simulink model "ardupilotsailboat"  (R2024a)
settings: Solver=ode15s  StartTime=0.0  StopTime=2  RelTol=1e-3
values from neighbouring files (symbols this model uses):
  Ixx = 1/120 * pi * rho * L * B * T * (4*T^2 + B^2)    (= 0.835683076278)    [parameterCalculations.m]
  Izz = 1/120 * pi * rho * L * B * T * (B^2 + L^2)    (= 1.17027496573)    [parameterCalculations.m]
  m = 2.7    [parameterCalculations.m]
  m11 = m*k11    [parameterCalculations.m]
  m22 = m*k22    [parameterCalculations.m]
  m24 = 0    [parameterCalculations.m]
  m26 = xb*m22    [parameterCalculations.m]
  m66 = k66*Izz    [parameterCalculations.m]
  Nr = -pi * T^2/L^2 * (0.25 +0.039 * B/T - 0.56 * B/L)    (= -0.104988463049)    [parameterCalculations.m]
  Nv = -pi * T^2/L^2 * (0.5 +2.4 * T/L)    (= -0.841300100031)    [parameterCalculations.m]
  Yv = -pi * T^2/L^2 * (1 +0.4 * CB * B/T)    (= -0.560439243466)    [parameterCalculations.m]
undefined symbols (not defined in the file or in its folder): Waypoints
libraries: cstblocks x6, simulink x4, vrlib x1
(part 2 of 2)

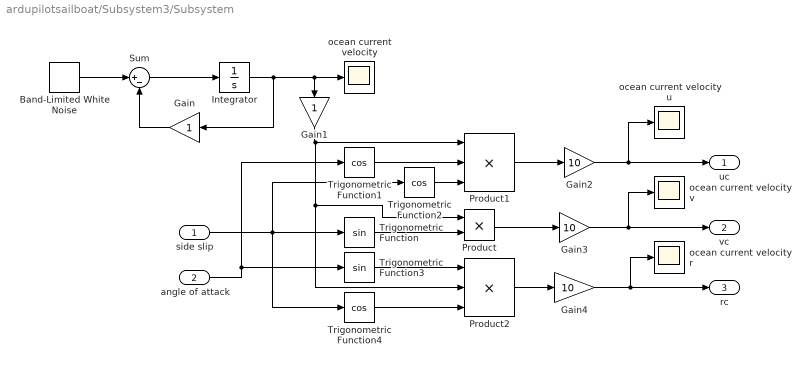
== system ardupilotsailboat/Subsystem3/Subsystem ==
  side slip : Inport
  angle of attack : Inport  Port=2
  Band-Limited White Noise : simulink/Sources/Band-Limited White Noise  Cov=[0.03]  Ts=1  seed=[23341]
  Gain : Gain
  Gain1 : Gain
  Gain2 : Gain  Gain=10
  Gain3 : Gain  Gain=10
  Gain4 : Gain  Gain=10
  Integrator : Integrator
  Product : Product
  Product1 : Product  Inputs=3
  Product2 : Product  Inputs=3
  Sum : Sum  Inputs=|+-
  Trigonometric Function : Trigonometry
  Trigonometric Function1 : Trigonometry  Operator=cos
  Trigonometric Function2 : Trigonometry  Operator=cos
  Trigonometric Function3 : Trigonometry
  Trigonometric Function4 : Trigonometry  Operator=cos
  ocean current velocity : Scope
  ocean current velocity r : Scope
  ocean current velocity u : Scope
  ocean current velocity v : Scope
  uc : Outport
  vc : Outport  Port=2
  rc : Outport  Port=3
  wires:
  Sum/1 -> Integrator/1
  Band-Limited White Noise/1 -> Sum/1
  Integrator/1 -> ocean current velocity/1, Gain1/1, Gain/1
  Gain/1 -> Sum/2
  Trigonometric Function/1 -> Product/2
  side slip/1 -> Trigonometric Function4/1, Trigonometric Function2/1, Trigonometric Function/1
  Product/1 -> Gain3/1
  Trigonometric Function2/1 -> Product1/3
  Trigonometric Function1/1 -> Product1/2
  Product1/1 -> Gain2/1
  Trigonometric Function3/1 -> Product2/1
  Trigonometric Function4/1 -> Product2/3
  angle of attack/1 -> Trigonometric Function3/1, Trigonometric Function1/1
  Product2/1 -> Gain4/1
  Gain1/1 -> Product1/1, Product2/2, Product/1
  Gain2/1 -> ocean current velocity u/1, uc/1
  Gain3/1 -> ocean current velocity v/1, vc/1
  Gain4/1 -> rc/1, ocean current velocity r/1

== matlab function ardupilotsailboat/MATLAB Function3 ==
  data: Xs output; delta_s input; wind_direction input; Ys output; Ks output; Ns output; awa output; wind_velocity input; psi input; u input; v input; r input; alpha_aw output; apparent_velocity output; V_awu output; V_awv output; L output; D output
function [Xs,Ys,Ks,Ns,awa,alpha_aw,apparent_velocity,V_awu,V_awv,L,D] = sailForce(delta_s,wind_direction,wind_velocity, psi, u, v,r)
%Parameters
rho_a = 1.2;
area_sail =0.38;

% CoE of the sail
xs = 0;
ys = 0;
zs = 0.6;
xm = 0;
xsm = 0; 
v_t = [wind_velocity*cos(wind_direction); wind_velocity*sin(wind_direction); 0 ];
R1 = [ cos(-psi) -sin(-psi) 0; sin(-psi) cos(-psi) 0; 0 0 1];
R2 = [ 1 0 0 ; 0 1 0; 0 0 1];
v_tb = R2*R1*v_t; % wind expressed in the body frame
V_in = [ u ; v ; 0 ];
V_awb = v_tb - V_in ;
V_awu = V_awb(1);
V_awv = V_awb(2);
V_aw = V_awu^2 + V_awv^2;
alpha_aw = atan2(real(V_awv),real(-V_awu));


% Apparent Wind Velocity
awa=alpha_aw;
apparent_velocity = sqrt(V_aw);

% Calculate Angle of Attack
alpha = awa+delta_s;


% Calculate Lift and Drag Force
[Cls,Cds] = sailcoef(alpha);
Ls = 0.5*rho_a*area_sail*(apparent_velocity)^2*Cls;
Ds = 0.5*rho_a*area_sail*(apparent_velocity)^2*Cds;

% Sail Force components
Xs =(Ls * sin(awa) - Ds * cos(awa));
Ys = (Ls * cos(awa) + Ds * sin(awa));
Ks = -zs *(Ls * cos(awa) + Ds * sin(awa));
Ns = (-Xs * xsm * sin(delta_s) +Ys*(xm-xsm*cos(delta_s)));
L = Ls*sin(awa);
D = -Ds*cos(awa);

function [Cls,Cds] = sailcoef(attack)
% generate a lookup table for the lift/drag coefficients for the sail
% and compute Cls/Cds from the lookup table using interpolation.

% lookup table
xdata = linspace(-pi,pi,73); % every 5 degrees
xdata = xdata/pi*180;

% lift curve
yldata = [fliplr([0 0.15 0.32 ...
    0.48 0.7 0.94 1.15 1.3 1.28 1.15 1.1 1.05 1 0.9 0.82 0.72 0.68 0.56 0.48 0.32 0.21 0.08 ...
    -0.06 -0.18 -0.3 -0.4 -0.53 -0.64 -0.72 -0.84 -0.95 -1.04 -1.1 -1.14 -1.08 -0.76 0])*(-1) ...
    [0.15 0.32 ...
    0.48 0.7 0.94 1.15 1.3 1.28 1.15 1.1 1.05 1 0.9 0.82 0.72 0.68 0.56 0.48 0.32 0.21 0.08 ...
    -0.06 -0.18 -0.3 -0.4 -0.53 -0.64 -0.72 -0.84 -0.95 -1.04 -1.1 -1.14 -1.08 -0.76 0]];

% drag curve
yddata = [fliplr([0.1 0.12 0.14 ...
    0.16 0.19 0.26 0.35 0.46 0.54 0.62 0.7 0.78 0.9 0.98 1.04 1.08 1.16 1.2 1.24 1.26 ...
    1.28 1.34 1.36 1.37 1.33 1.31 1.28 1.26 1.25 1.2 1.1 1.04 0.88 0.8 0.64 0.38 0.1])...
    [0.12 0.14 ...
    0.16 0.19 0.26 0.35 0.46 0.54 0.62 0.7 0.78 0.9 0.98 1.04 1.08 1.16 1.2 1.24 1.26 ...
    1.28 1.34 1.36 1.37 1.33 1.31 1.28 1.26 1.25 1.2 1.1 1.04 0.88 0.8 0.64 0.38 0.1]];

% fit the input angle of attack into the interval [-pi,pi]
if attack > pi
    attack = mod(attack+pi,2*pi) - pi;
else
    if attack < -pi
        attack = mod(attack-pi,-2*pi) + pi;
    end
end

% interpolation
attack = attack/pi*180;
Cls = interp1(xdata,yldata,attack,'pchip');
Cds = interp1(xdata,yddata,attack,'pchip');

== matlab function ardupilotsailboat/MATLAB Function4 ==
  data: r input; u input; Xr output; v input; Yr output; Kr output; Nr output; delta_r input; delta_r output; alpha_a output; p input; phi input; lift_force output; drag_force output
function [Xr, Yr, Kr, Nr, delta_r, alpha_a, lift_force, drag_force] = rudderForce(r, u, v, delta_r, p, phi)
%Parameters
rudder_width = 4;
rudder_length = 20;
rho_w = 1025;
area = rudder_length * rudder_width * 10^(-4);
velocity = sqrt(v^2+u^2);
yr = 0;
xr = 0.55;
zr = 0.2;
zeta_r =1; % Rudder Efficiency
d_r = 0.2; % Rudder Draft
% Calculate Angle of Attack
v_aru = -u + r*yr;
v_arv = -v-r*xr;
alpha_ar = atan2(real(v_arv),real(v_aru));
alpha_a = alpha_ar - delta_r;

% Lift and Drag Coeff
[lc, dc] = ruddercoef(alpha_a);
dc = dc+lc^2*area*(pi*2*zeta_r*d_r^2);

% Calculate Lift and Drag Force
lift_force = 0.5 * rho_w * area * lc * (v_aru^2+v_arv^2) ;
drag_force = 0.5 * rho_w * area * dc * (v_aru^2+v_arv^2) ;

Xr = (lift_force * sin(alpha_ar) - drag_force * cos(alpha_ar));
Yr = (lift_force * cos(alpha_ar) + drag_force * sin(alpha_ar))*cos(phi);
Kr = zr * ( -lift_force * cos(alpha_ar) - drag_force * sin(alpha_ar));
Nr = xr * (lift_force * cos(alpha_ar) + drag_force * sin(alpha_ar))*cos(phi);
Nr = Nr*1.25;


function [Clr,Cdr] = ruddercoef(attack)
% generate a lookup table for the lift/drag coefficients for the sail
% and compute Cls/Cds from the lookup table using interpolation.

% lookup table
xdata = linspace(-pi,pi,73); % every 5 degrees
xdata = xdata/pi*180;

% lift curve
yl = fliplr([0 0.42 0.73 ...
    0.95 1.1 1.165 1.18 1.155 1.12 1.065 1 0.92 0.83 0.72 0.62 0.48 0.33 0.16])*(-1);
yldata = [fliplr([0 0.42 0.73 ...
    0.95 1.1 1.165 1.18 1.155 1.12 1.065 1 0.92 0.83 0.72 0.62 0.48 0.33 0.16 0 yl])*(-1) ...
    [0.42 0.73 ...
    0.95 1.1 1.165 1.18 1.155 1.12 1.065 1 0.92 0.83 0.72 0.62 0.48 0.33 0.16 0 yl]];

% drag curve
yd = fliplr([0 0.03 0.06 ...
    0.1 0.17 0.3 0.48 0.74 0.98 1.18 1.34 1.5 1.65 1.76 1.89 1.97 2.01 2.05]);
yddata = [fliplr([0 0.03 0.06 ...
    0.1 0.17 0.3 0.48 0.74 0.98 1.18 1.34 1.5 1.65 1.76 1.89 1.97 2.01 2.05 2.08 yd])...
    [0.03 0.06 ...
    0.1 0.17 0.3 0.48 0.74 0.98 1.18 1.34 1.5 1.65 1.76 1.89 1.97 2.01 2.05 2.08 yd]];

% fit the input angle of attack into the interval [-pi,pi]
if attack > pi
    attack = mod(attack+pi,2*pi) - pi;
else
    if attack < -pi
        attack = mod(attack-pi,-2*pi) + pi;
    end
end

% interpolation
attack = attack/pi*180;
Clr = interp1(xdata,yldata,attack,'pchip');
Cdr = interp1(xdata,yddata,attack,'pchip');

== matlab function ardupilotsailboat/MATLAB Function5 ==
  data: r input; u input; Xk output; v input; Yk output; Kk output; Nk output; phi input
function [Xk,Yk,Kk,Nk] = keelForce(r,u,v,phi)
%Parameters
keel_width = 8;
keel_length = 45;
rho_w = 1025;
area = keel_width * keel_length * 10^(-4);
velocity = sqrt(v^2+u^2);
l3 = 0.1;
h2 =0.275;
yk=0;
xk=0;
zk=0.25;
zeta_r = 1;
d_r = 0.4;
% Calculate Angle of Attack
v_aku = -u + r*yk;
v_akv = -v - r*xk + 0*zk;
alpha_ak = atan2(real(v_akv),real(-v_aku));
alpha = alpha_ak;

% Lift and Drag Coeff
[lc, dc] = keelcoef(alpha);
dc = dc+lc^2*area*(pi*2*zeta_r*d_r^2);

% Calculate Lift and Drag Force
lift_force = 0.5 * rho_w * area * lc * (v_aku^2+v_akv^2);
drag_force = 0.5 * rho_w * area * dc * (v_aku^2+v_akv^2);

Xk = (-lift_force * sin(alpha_ak) + drag_force * cos(alpha_ak));
Yk = (-lift_force * cos(alpha_ak) - drag_force * sin(alpha_ak))*cos(phi);
Kk = (lift_force*cos(alpha_ak)+drag_force*sin(alpha_ak))*zk;
Nk = (-(lift_force*cos(alpha_ak)-drag_force*sin(alpha_ak))*xk)*cos(phi);




%------------------------------------------------------------------------------------------------------------------------------
function [Clk,Cdk] = keelcoef(attack)
% generate a lookup table for the lift/drag coefficients for the sail
% and compute Cls/Cds from the lookup table using interpolation.

% lookup table
xdata = linspace(-pi,pi,73); % every 5 degrees
xdata = xdata/pi*180;

% lift curve
yl = fliplr([0 0.425 0.74 ...
    0.94 1.1 1.17 1.19 1.16 1.12 1.07 0.99 0.92 0.84 0.74 0.63 0.49 0.345 0.185])*(-1);
yldata = [fliplr([0 0.425 0.74 ...
    0.94 1.1 1.17 1.19 1.16 1.12 1.07 0.99 0.92 0.84 0.74 0.63 0.49 0.345 0.185 0 yl])*(-1) ...
    [0.425 0.74 ...
    0.94 1.1 1.17 1.19 1.16 1.12 1.07 0.99 0.92 0.84 0.74 0.63 0.49 0.345 0.185 0 yl]];

% drag curve
yd = fliplr([0 0.04 0.07 ...
    0.1 0.17 0.3 0.49 0.76 0.98 1.19 1.34 1.5 1.65 1.77 1.88 1.96 2.01 2.05]);
yddata = [fliplr([0 0.04 0.07 ...
    0.1 0.17 0.3 0.49 0.76 0.98 1.19 1.34 1.5 1.65 1.77 1.88 1.96 2.01 2.05 2.09 yd])...
    [0.04 0.07 ...
    0.1 0.17 0.3 0.49 0.76 0.98 1.19 1.34 1.5 1.65 1.77 1.88 1.96 2.01 2.05 2.09 yd]];

% fit the input angle of attack into the interval [-pi,pi]
if attack > pi
    attack = mod(attack+pi,2*pi) - pi;
else
    if attack < -pi
        attack = mod(attack-pi,-2*pi) + pi;
    end
end

% interpolation
attack = attack/pi*180;
Clk = interp1(xdata,yldata,attack,'pchip');
Cdk = interp1(xdata,yddata,attack,'pchip');


%------------------------------------------------------------------------------------------------------------------------------
function F = resistancehull(alpha_a)

xdata = linspace(0,6,13); % every 0.5m/s
ydata = [0 0.15 0.35 0.5 0.675 0.825 1.175 1.4 2 4.85 9.85 18.46 27.5]*1000;

% interpolation
if alpha_a <= 6
    F = interp1(xdata,ydata,alpha_a,'pchip');
else
    F = interp1(xdata,ydata,alpha_a,'pchip','extrap');
end

== matlab function ardupilotsailboat/MATLAB Function6 ==
  data: r input; u input; Xh output; v input; Yh output; Kh output; Nh output; Frh output; phi input; alpha_ah output
function [Xh,Yh,Kh,Nh,Frh,alpha_ah] = hullForce(r,u,v,phi)
yh = 0;
zh = 0.1;
xh = 0;
B = 0.125;
rho = 1025;
L = 0.95;
Lwl =0.85;
g = 9.81;
delta =  4*pi * (((0.475*0.0625)^(1.6)+(0.475*0.1)^(1.6)+(0.0625*0.1)^(1.6))/(3))^(1/1.6);
% from the hull
v_ahu = -u + r*yh;
v_ahv = (-v-r*xh + 0*zh)/cos(0);
v_ah = sqrt(v_ahu^2 + v_ahv^2);
alpha_ah = atan2(real(v_ahv),real(v_ahu));
%Frh = resistancehull(u);
Re = (abs(v_ahu)*Lwl)/(0.00000010034);
Cf = 0.075 / (log(Re)-2)^2;
Frh = 0.5 * rho * u^2 * Cf * (delta);

Xh = Frh;

Yh = -Frh*sin(alpha_ah)*cos(phi);

if abs(Yh)>15
    if Yh >0
        Yh=15;
    else
        Yh = -15;
    end
end
Kh = Frh*sin(alpha_ah)*cos(phi)*zh;

if abs(Kh)>15
    if Kh >0
        Kh=15;
    else
        Kh = -15;
    end
end
Nh = -Frh*sin(alpha_ah)*cos(0)*xh;
%D_hull = [Frh*cos(alpha_ah);-Frh*sin(alpha_ah)*cos(phi); Frh*sin(alpha_ah)*cos(phi)*par.zh; -Frh*sin(alpha_ah)*cos(phi)*par.xh];


function F = resistancehull(alpha_a)

xdata = linspace(0,2.6,13); % every 0.5m/s
ydata = [0 6.0018e-04 0.0039*0.0039 0.0127*0.0127 0.0306*0.0306 0.0625*0.0625 0.1157*0.1157 0.2002*0.2002 0.3304*0.3304 0.5274*0.5274 0.8219*0.8 1.2606*0.9 1.9151];

% interpolation
if alpha_a <= 1.3
    F = interp1(xdata,ydata,alpha_a,'pchip');
else
    F = interp1(xdata,ydata,alpha_a,'pchip','extrap');
end

== matlab function ardupilotsailboat/Subsystem8/MATLAB Function19 ==
  data: y output; v input; u input; y1 output
function [y,y1]     = beta(v,u)
% Beta Reference Angle
y=0;
y1 = real(asin(complex(v/sqrt(v^2+u^2))));

== matlab function ardupilotsailboat/MATLAB Function1 ==
  data: y output; psi input; currentState input; nextState output
function [y,nextState]      = zigzagPsi(psi,currentState)

switch currentState
    case 0
        if(psi>(20/180*pi))
            nextState=1;
        else
            nextState=0;
        end
        y=21/180*pi;
    case 1 
        if (psi<-(20/180*pi))
            nextState=0;
        else
            nextState=1;
        end
        y=-21/180*pi;
    otherwise
    y=0;
    nextState=0;
end

== matlab function ardupilotsailboat/Subsystem7/MATLAB Function1 ==
  data: roll_angle input; current_state input; t input; sail_angle output; t_prev input; next_state output; t_state_change output; apparent_wind_angle input
%%%%%%%%%%%%%%%%%%%%%%%%%%%%%%%%%%%%%%%%%%%%%%%%%%%%%%%%%%%%%%
%SAIL CONTROLLER
%%%%%%%%%%%%%%%%%%%%%%%%%%%%%%%%%%%%%%%%%%%%%%%%%%%%%%%%%%%%%%
function [sail_angle,next_state,t_state_change]  = sailAngle(roll_angle,current_state,t,t_prev,apparent_wind_angle)
switch(current_state)
    case 0
        sail_angle = 60;
        if (t - t_prev) >0.5
            if roll_angle <12
               next_state = 1;
               t_state_change = t;
            else
                next_state =0;
                t_state_change = t_prev;
            end
        else
            next_state = 0;
            t_state_change = t_prev;
        end
    case 1
        sail_angle = 45;
        if (t - t_prev) >0.5
            if roll_angle > 12
                next_state = 0;
                t_state_change = t;
            elseif roll_angle <8
                next_state =2;
                t_state_change = t;
            else
                next_state =1;
                t_state_change = t_prev;
            end
        else
            next_state =1;
            t_state_change = t_prev;
        end
    case 2
        sail_angle = 30;
        if (t - t_prev) >0.5
            if roll_angle > 12
                next_state = 1;
                t_state_change = t;
            else 
                next_state =2;
                t_state_change = t_prev;
            end
        else
            next_state =2;
            t_state_change = t_prev;
        end
    otherwise
        sail_angle = 60;
        next_state=0;
        t_state_change = t;
end
if apparent_wind_angle >0 
    sail_angle = -sail_angle;
end

== matlab function ardupilotsailboat/MATLAB Function7 ==
  data: y output; r input; currentState input; nextState output
function [y,nextState]      = zigzag(r,currentState)
% Beta Reference Angle

switch currentState
    case 0
        if(r==1)
        nextState=1;
        else 
            nextState=0;
        end
        y=10/180*pi;
    case 1
        if(r==1)
        nextState=0;
        else 
            nextState=1;
        end
        y=-10/180*pi;
    otherwise
        y=10/180*pi;
        nextState=0;
end

== matlab function ardupilotsailboat/Subsystem1/MATLAB Function1 ==
  data: awa input; psi input; y output
function y = controlAngle(awa,psi)
if psi<-2*pi
    psi=psi+2*pi;
end
if psi>2*pi
    psi=psi-2*pi;
end


y = awa+psi;

== matlab function ardupilotsailboat/MATLAB Function8 ==
  data: y output; psi input; state input
function y      = zigzagPsi(psi,state)
% Beta Reference Angle
if psi<-10 && state == 1
    y=1;
elseif psi>10 && state == 0
    y=1;
else 
    y=0;
end

== matlab function ardupilotsailboat/Subsystem1/MATLAB Function2 ==
  data: x1 input; y1 input; u input; y output; us input; u1 output
function [y,u1] = controlAngle(x1,y1,u,us)
ys=0;
if x1>=0 && y1>=0
    ys=u;
elseif x1>=0 && y1<=0
        ys=pi-u;
elseif x1==0 && y1>0
        ys=-pi;
elseif x1==0 && y1<0
        ys=pi;
elseif y1==0 && x1>0
        ys=pi/2;
elseif y1==0 && x1<0
        ys=-pi/2;
elseif x1<0 && y1>0
    ys=-u-pi;
elseif x1<0 && y1<0
    ys=-pi+u;
else
    ys=u;
end
if (ys-us)<-pi
    %y = ys+2*pi;
elseif (ys-us)>pi
   % y=ys-2*pi;
else
    y=ys;
end
y=ys;
u1=u;

== matlab function ardupilotsailboat/Subsystem1/MATLAB Function13 ==
  data: u input; v input; psi input; psiTrack input; uTrack output; trackDistanceToWaypoint input; closeToWaypoint output
function[uTrack,closeToWaypoint]   = trackVelocity(u,v,psi,psiTrack,trackDistanceToWaypoint)
% Calculate track velocity of sailboat

% Velocity Vector
U = sqrt(u^2+v^2);
psiU = atan(v/u);

psiA = psi + psiU;

uTrack = U * cos(psiTrack + psiA);
closeToWaypoint = 0;
if (trackDistanceToWaypoint/abs(uTrack))<10
    closeToWaypoint = 1;
end

== matlab function ardupilotsailboat/Subsystem1/MATLAB Function10 ==
  data: state input; y output
function y = stopSimulation(state)
if state== 3
    y=1;
else
    y=0;
end

== matlab function ardupilotsailboat/Subsystem1/MATLAB Function14 ==
  data: closeToWaypoint input; switchTack output; tacking input; waypointApproach input; psiOffset output
function [switchTack, psiOffset]   = orientSailboat(closeToWaypoint,tacking, waypointApproach)
% Orientate sailboat so that it passes waypoint with its port side
% Port: 0 
% Starboard: 1 
switchTack=0;
psiOffset=0;
if tacking == 1 || tacking == 2 || tacking == 3
        if closeToWaypoint==1
                switchTack = 1;
        else
            switchTack=0;
        
        end
        psiOffset=0;
elseif tacking==0
    if waypointApproach == 0
        psiOffset=10/180*pi;

    else
        psiOffset = -10/180*pi;
    end
    
end

== matlab function ardupilotsailboat/MATLAB Function2 ==
  data: t input; amplitude output; gust_direction input; direction output
function [amplitude, direction] = windModel(t,gust_direction)
% Initialize Parameters
mean_speed = 5; %m/s
z = -0.5; % height of centre of effort points on sail:
n = 0.468; % constant
f = 0:0.1:0.4;  % frequencies
distribution = 0:2*pi/5:2*pi-2*pi/5;
upsilon = 1:1:5;
upsilon(1) = distribution(1)*2*pi;    % phase distribution
upsilon(2) = distribution(2)*2*pi; 
upsilon(3) =distribution(3)*2*pi; 
upsilon(4) =distribution(4)*2*pi; 
upsilon(5) =distribution(5)*2*pi; 
mean_direction = 5*pi/6;
amplitude_gust = 1:1:5;
amplitude_comp = 1:1:5;
for i=1:1:length(f)
    x_z = 172*f(i)*(-z)^(2/3)*(mean_speed)^(-0.75);
    S = 320 * (mean_speed^2 * -z) / (1 + x_z^n )^(5/(3*n));
    amplitude_gust(i) = sqrt(2*S*f(i))* cos(2*pi*f(i)*t + upsilon(i));
end
for i=1:1:length(amplitude_gust)
    amplitude_comp(i) = amplitude_gust(i);
end
amplitude = (amplitude_comp(1) + amplitude_comp(2) + amplitude_comp(3) + amplitude_comp(4) + amplitude_comp(5))/5 ;
direction =  gust_direction;

== matlab function ardupilotsailboat/Subsystem1/MATLAB Function16 ==
  data: x input; y output; y input; x1 input; y1 input
function y = trackDistance(x,y,x1,y1)
y = sqrt((x-x1)^2+(y-y1)^2);

== matlab function ardupilotsailboat/MATLAB Function9 ==
  data: y output; t input; currentState input; nextState output
function [y,nextState]      = zigzag(t,currentState)
% Beta Reference Angle

switch currentState
    case 0
        if (t<0.3)
            nextState=0;
            y= 10/180*pi;
        else
            nextState=1;
             y=-10/180*pi;
        end
    case 1
         if (t<0.95)
            nextState=1;
            y= -10/180*pi;
        else
            nextState=2;
             y=10/180*pi;
         end
    case 2
         if (t<1.55)
            nextState=2;
            y=10/180*pi;
        else
            nextState=3;
             y=-10/180*pi;
         end
    case 3
         if (t<2.25)
            nextState=3;
            y= -10/180*pi;
        else
            nextState=4;
             y=10/180*pi;
         end
    case 4
         if (t<2.85)
            nextState=4;
            y= 10/180*pi;
        else
            nextState=5;
             y=-10/180*pi;
         end
   case 5
         if (t<3.6)
            nextState=5;
            y= -10/180*pi;
         else 
             y=0;
             nextState=6;
         end
  case 6
         y=0;
         nextState=6;
  otherwise
        y=10/180*pi;
        nextState=0;
end

== matlab function ardupilotsailboat/Subsystem1/MATLAB Function11 ==
  data: xw input; yw input; xs input; p_w output; ys input; xcw input; ycw input; theta output; pwc input; pwn output; thetaP input
function [p_w,theta,pwn] = passedWaypoint(xw,yw,xs,ys,xcw,ycw,pwc,thetaP)
% Checking is sailboat has passed waypoint while sailing into the wind
switch pwc
    case 0
        if (ys-ycw)~= 0 
            theta = atan(abs(xs-xcw)/abs(ys-ycw));
            pwn=1;
        else 
            pwn=0;
            theta=0;
        end
    case 1
        theta=thetaP;
        pwn=1;
    otherwise
    theta=thetaP;
    pwn=0;
end

p_w=0;
if xw>0 
% Angle between sail
    if (xcw-xs)<0 
        % Waypoint passed in x positive
        p_w=1;
        if(ycw-ys)<0
            % Waypoint passed in both x and y positive direction
            theta = pi + theta;
        else
            % Waypoint passed in positive x and negative y
            theta = -theta;
        end
    end 
else
    if(xcw-xs)>0 
        % Waypoint passed in x negative
        p_w=1;
        if(ycw-ys)>0
           % Waypoint passed in both x and y negative direction
        else
           % Waypoint passed in negative x and positive y
           theta= pi - theta;
        end
   end
end

if p_w==1
    
end

== matlab function ardupilotsailboat/Subsystem1/MATLAB Function12 ==
  data: xs input; ys input; x input; y input; dist input; dist output
function dist   = travelDistance(xs,ys,x,y,dist)
% Distance Sailboat travelled

dist = dist + sqrt((xs-x)^2+(ys-y)^2);

== matlab function ardupilotsailboat/Subsystem1/MATLAB Function18 ==
  data: angle input; nextState output; currentState input
function nextState    = tack_Side(angle,currentState)
% Calculate when to tack back to waypoint

switch currentState
    case 1
        % In zone 1 can go to zone 2 and 4
        if angle < 0
            nextState=4;
        elseif angle > 15
            nextState=2;
        else 
            nextState=1;
        end
    case 2
       % In zone 2 can go to zone 3 and 1
        if angle < 15
            nextState=1;
        elseif angle > 30
            nextState=3;
        else 
            nextState=2;
        end
    case 3
        % In zone 3 can go to zone 2
        if angle < 30
            nextState=2;
        else 
            nextState=3;
        end
    case 4
       % In zone 4 can go to zone 5 and 1
        if angle > 0
            nextState=1;
        elseif angle < -15
            nextState=5;
        else 
            nextState=4;
        end
    case 5
       % In zone 5 can go to zone 6 and 4
        if angle < -30
            nextState=6;
        elseif angle >-15
            nextState=4;
        else
            nextState=5;
        end
    case 6
        % In zone 6 can go to zone 5
        if angle > -30
            nextState=5;
        else 
            nextState=6;
        end
    otherwise
        nextState=1;

end

== matlab function ardupilotsailboat/Subsystem1/MATLAB Function3 ==
  data: pathTrajectory input; y output; tack input; tackDistance output; tackLeft output; tackRight output; AWA input; xtrack input; nextTackType output; indirectTackSide input; zone input; currentTackType input; currentState output; noGoAngle input; tackType input; XtrackDistance input; passedWaypoint input; pwTrajectory input; switchSide input; closeToWay input; psiOffset input; Beta input
function [y,tackDistance, tackLeft,tackRight,nextTackType,currentState]  = headingController(pathTrajectory,tack,AWA,xtrack,indirectTackSide,zone,currentTackType,noGoAngle,tackType,XtrackDistance,passedWaypoint,pwTrajectory,switchSide,closeToWay,psiOffset,Beta)
% Heading State Machine

% Type of Tacks
% Direct = 1
% Indirect = 2
% Zones = 3

tackDistance = XtrackDistance;
if tack==0 && passedWaypoint==0
    currentState = 0;
elseif passedWaypoint==1 && (tackType==1 || tackType==2) 
    currentState = 4;
else
    % Switch between Direct and Indirect Tack and Zone Tack
    currentState = tackType;
end
switch currentState
    % Normail State 
    case 0
        y = pathTrajectory;
        nextTackType=1;
        tackLeft=0;
        tackRight=0;
    % Direct Tacking State
    case 1
       switch currentTackType
           case 1
               y=AWA+noGoAngle+Beta;
               tackRight=1;
               tackLeft=0;
               if(xtrack>tackDistance)
                   nextTackType=0;
               else
                   nextTackType=1;
               end
               
           case 0 
               y=AWA-noGoAngle+Beta;
               tackRight=0;
               tackLeft=1;
               if (xtrack<-tackDistance)
                   nextTackType=1;
               else 
                   nextTackType=0;
               end
           otherwise
               nextTackType=1;
               y=AWA+45;
               tackLeft=1;
               tackRight=0;
       end
    
    % Indirect Tacking State
    case 2
        if indirectTackSide==0
             y=AWA*180/pi+noGoAngle;
        else
             y=AWA*180/pi-noGoAngle;
        end
        nextTackType=1;
        tackLeft=0;
        tackRight=0;

    % Zone Tacking State
    case 3
        switch zone
            case 1
                if currentTackType==0
                    tackLeft=1;
                    tackRight=0;
                    y=AWA*180/pi-noGoAngle;
                    nextTackType=0;
                else
                    tackLeft=0;
                    tackRight=1;
                    y=AWA*180/pi+noGoAngle;
                    nextTackType=1;
                end

            case 2
                if currentTackType==0
                    tackLeft=1;
                    tackRight=0;
                    y=AWA*180/pi-noGoAngle;
                    nextTackType=0;
                else
                    tackLeft=0;
                    tackRight=1;
                    y=AWA*180/pi+noGoAngle;
                    nextTackType=1;
                end

            case 3
                % If boat is forced in zone 3 sail past lay lines and only
                % when one has passed the lay lines sail to waypoint
                y = pathTrajectory;
                tackLeft=1;
                nextTackType=0;
                tackRight=0;
            
            case 4
                if currentTackType==0
                    tackLeft=1;
                    tackRight=0;
                    y=AWA*180/pi-noGoAngle;
                    nextTackType=0;
                else
                    tackLeft=0;
                    tackRight=1;
                    y=AWA*180/pi+noGoAngle;
                    nextTackType=1;
                end

            case 5
                if currentTackType==0
                    tackLeft=1;
                    tackRight=0;
                    y=AWA*180/pi-noGoAngle;
                    nextTackType=0;
                else
                    tackLeft=0;
                    tackRight=1;
                    y=AWA*180/pi+noGoAngle;
                    nextTackType=1;
                end

            case 6
                % Same as zone 3 just opposite tack
                y = pathTrajectory;
                tackLeft=0;
                nextTackType=1;
                tackRight=1;

            otherwise
                y = pathTrajectory;
                nextTackType=0;
                tackLeft=1;
                tackRight=0;
        end

    case 4
        y = pwTrajectory;
        tackLeft=0;
        nextTackType=1;
        tackRight=1;

    otherwise
        y=0;
        nextTackType=2;
        tackLeft=0;
        tackRight=0;

end


if currentState==3
    if tackLeft==1
         y=AWA*180/pi-noGoAngle;
         nextTackType=0;
    else
         y=AWA*180/pi+noGoAngle;
         nextTackType=1;
    end
end
if currentState~=0
    if switchSide==1 && closeToWay==1
       nextTackType=1;
    end
end

== matlab function ardupilotsailboat/Subsystem1/MATLAB Function4 ==
  data: R input; nextState output; currentWaypoint output; currentState input
function [nextState,currentWaypoint]  = wayPointController(R,currentState)
% Waypoint switching
% With each added waypoint another case should be added
switch currentState
    % First waypoint
    case 0
        % Check if waypoint lies within radius of acceptance
        if(R==1)
            % Switch current Waypoint to next waypoint
            nextState=1;
            currentWaypoint=1;
        % Waypoint not reached
        else
            nextState=0;
            currentWaypoint=0;
        end
    case 1
        % Check if waypoint lies within radius of acceptance
        if(R==1)
            % Switch current Waypoint to next waypoint
            nextState=2;
            currentWaypoint=2;
       % Waypoint not reached
       else
            nextState=currentState;
            currentWaypoint=1;
       end
    case 2
       % Check if waypoint lies within radius of acceptance
       if(R==1)
            % Switch current Waypoint to next waypoint
            nextState=3;
            currentWaypoint=3;
       % Waypoint not reached
       else
            nextState=currentState;
            currentWaypoint=2;
       end
     case 3
       % Check if waypoint lies within radius of acceptance
       if(R==1)
            % Switch current Waypoint to next waypoint
            nextState=4;
            currentWaypoint=4;
       % Waypoint not reached 
       else
            nextState=currentState;
            currentWaypoint=3;
       end
     case 4
       % Check if waypoint lies within radius of acceptance
       if(R==1)
            % Switch current Waypoint to next waypoint
            nextState=5;
            currentWaypoint=5;
       % Waypoint not reached
       else
            nextState=currentState;
            currentWaypoint=4;
       end
       case 5
       % Check if waypoint lies within radius of acceptance
       if(R==1)
            % Switch current Waypoint to next waypoint
            nextState=6;
            currentWaypoint=6;
       % Waypoint not reached
       else
            nextState=currentState;
            currentWaypoint=5;
       end
       case 6
       % Check if waypoint lies within radius of acceptance
       if(R==1)
            % Switch current Waypoint to next waypoint
            nextState=0;
            currentWaypoint=0;
       % Waypoint not reached
       else
            nextState=currentState;
            currentWaypoint=6;
       end
    otherwise
        nextState=0;
        currentWaypoint=0;
end

== matlab function ardupilotsailboat/Subsystem1/MATLAB Function5 ==
  data: xWaypoint input; yWaypoint input; xBoat input; yBoat input; R input; acceptance output; dist output; ltrack input
function [acceptance,dist]   = circleOfAcceptanceController(xWaypoint,yWaypoint,xBoat,yBoat,R,ltrack)
dist = sqrt((abs(xWaypoint-xBoat))^2+(abs(yWaypoint-yBoat))^2);
    if (sqrt((abs(xWaypoint-xBoat))^2+(abs(yWaypoint-yBoat))^2)<R)
        acceptance=1;
    else
        acceptance=0;
    end
    if ltrack <0 
        acceptance =1;
    end

end

== matlab function ardupilotsailboat/Subsystem1/MATLAB Function6 ==
  data: xw input; yw input; xwp input; y output; ywp input
function y  = distanceToWaypoint(xw,yw,xwp,ywp)
% Calculate distance to waypoint
y = (sqrt((ywp-yw)^2+(xwp-xw)^2))/2;

== matlab function ardupilotsailboat/Subsystem1/MATLAB Function7 ==
  data: wind input; tack output; psi input; awa output; currentState input; nextState output
function [tack,awa,nextState]   = apparentWindAngle(wind,psi,currentState)
% Calculate Apparent Wind Angle

if psi> 180
    psi= psi-2*180;
else
    if psi<-180
    psi=psi+2*180;
    end
end
awa = psi-wind-180;

if awa > 180
    awa=awa-360;
elseif awa <-180
    awa=awa+360;
end
switch currentState
    case 0 
        if abs(awa)<45
           tack = 1;
           nextState = 1;
        else
            tack = 0;
            nextState = 0;
        end
    case 1
        if abs(awa)>60
           tack = 0;
           nextState = 0;
        else
            tack = 1;
            nextState = 1;
        end
    otherwise
        nextState = 0;
        tack = 0;
end

== matlab function ardupilotsailboat/Subsystem1/MATLAB Function8 ==
  data: x1 input; y1 input; u input; y output; us input
function y = controlAngle(x1,y1,u,us)
ys=0;
if x1>=0 && y1>=0
    ys=u;
elseif x1>=0 && y1<=0
        ys=pi-u;
elseif x1==0 && y1>0
        ys=0;
elseif x1==0 && y1<0
        ys=pi;
elseif y1==0 && x1>0
        ys=pi/2;
elseif y1==0 && x1<0
        ys=-pi/2;
elseif x1<0 && y1>0
    ys=-u;
elseif x1<0 && y1<0
    ys=-pi+u;
else
    ys=u;
end
if (ys-us)<-pi
    y = ys+2*pi;
elseif (ys-us)>pi
    y=ys-2*pi;
else
    y=ys;
end

== matlab function ardupilotsailboat/Subsystem1/MATLAB Function9 ==
  data: angle output; dist input; xtrack input; currentState input; tack output; nextState output; windDirection input; wayPointHeading input
function [angle,tack,nextState]  = tackAngle(dist,xtrack,currentState,windDirection,wayPointHeading)
% Calculate when to tack back to waypoint
if dist ~= 0
    angle = atan(xtrack/dist);
else
    angle=0;
end

if windDirection > pi
    windDirection = windDirection - pi;
else
    if windDirection < -pi
        windDirection = windDirection + pi;
    end
end

if wayPointHeading > pi
    wayPointHeading = wayPointHeading - pi;
else
    if wayPointHeading < -pi
        wayPointHeading = wayPointHeading + pi;
    end
end

angle = angle * (180/pi) - (windDirection-wayPointHeading);

% tack == 0 is left tack
% tack == 1 is right tack
switch currentState
    case 0
        tack=0;
        if angle>=45
            nextState=1;
        else
            nextState=0;
        end
    case 1
        tack=1;
        if angle<=-45
            nextState=0;
        else
            nextState=1;
        end

    otherwise
        tack=0;
        nextState=0;

end

== matlab function ardupilotsailboat/Subsystem1/MATLAB Function15 ==
  data: u input; v input; Beta output
function Beta    = trackVelocity(u,v)
% Calculate track velocity of sailboat

% Velocity Vector
U = sqrt(u^2+v^2);
Beta = asin(v/U);

== matlab function ardupilotsailboat/Subsystem2/MATLAB Function ==
  data: u input; y output
function y = fcn(u)
if u>0
    y = -0.035
else 
    y=0;
end

== matlab function ardupilotsailboat/Subsystem8/MATLAB Function ==
  data: u input; y output; max input
function y = fcn(u,max)
if u>max
    u=max;
else 
    if u<-max
        u=-max;
    end
end
y = u;

== matlab function ardupilotsailboat/Subsystem7/MATLAB Function ==
  data: u input; y output; max input; min input
function y = fcn(u,max,min)
if u>max
    u=max;
else 
    if u<min
        u=min;
    end
end
y = u;

== matlab function ardupilotsailboat/Subsystem8/MATLAB Function1 ==
  data: u input; y output; max input
function y = fcn(u,max)
if u>max
    u=max;
else 
    if u<-max
        u=-max;
    end
end
y = u;

== matlab function ardupilotsailboat/Subsystem3/MATLAB Function14 ==
  data: beta input; wu output; wv output; wr output; t input
function [wu,wv,wr] = WaveForcesandMoments(beta,t)
% Water density (kg/m^2)
rho = 1025;

% Gravity (m/s^2)
g = 9.81;

% Vessel size (m)
L = 1;
B = 0.125;
T = 0.4;

% Vessels Heading

% Wave Specifications
% amplitude(m)
Ai = 2;
% length(m)
lamdai = 1;
% encounter frequency (rads)
omegai = 0.4;
% random phase (rads)
phii = -pi;

% Wave Component
waveC = Ai * (2*pi)/lamdai * sin(omegai*t + phii);

% u Component
wu = (10^(-6)) * rho * g * B * L * T * cos(beta) * waveC;

% v Component
wv = (10^(-6)) * rho * g * B * L * T * sin(beta) * waveC;

% r Component
wr = (10^(-6)) * 1/24 * rho * g * B * L * (L^2 - B^2) * sin(2*beta) * waveC^2;

== matlab function ardupilotsailboat/Subsystem3/MATLAB Function15 ==
  data: windDirect input; wi_u output; wi_v output; wi_r output; V_w input; psi input; u input; v input
function [wi_u,wi_v,wi_r] = WindForcesandMoments(windDirect,V_w,psi,u,v)
% Air density (kg/m^2)
rho = 1.225;

% Ship Size
L = 2;
B = 0.125;
T = 0.4;

% centroids above the water line of the frontal and lateral projected areas
H_fw = T - 1.2;
H_lw = T - 1.2;
A_fw = B * H_fw;
A_lw = L * H_lw;


% Symmetrical Ship Coeff
c_x = 0.7;
c_y = 0.825;
c_r = 0.125;

% Wind Velocities in x- and y-coordinates
u_w = V_w * cos(windDirect - psi);
v_w = V_w * sin(windDirect - psi);

% Relative wind velocities
u_rw = u - u_w;
v_rw = v - v_w;

% Relative Wind Velocity and direction
V_rw = sqrt(u_rw^2 + v_rw^2);
gamma_rw = -atan(v_rw/u_rw);

% Wind Coeff
C_x = -c_x * cos(gamma_rw);
C_y = c_y * sin(gamma_rw);
C_r = c_r * sin(2*gamma_rw);

% Wind Forces and Moments
wi_u = 0.5 * rho * V_rw *  C_x * A_fw * 10^(-2);
wi_v = 0.5 * rho * V_rw *  C_y * A_lw * 10^(-2);
wi_r = 0.5 * rho * V_rw *  C_r * A_lw * 10^(-2);
